simulink model "HVDCThyristorBased"  (R2024b)
settings: Solver=FixedStepDiscrete  StartTime=0.0  StopTime=2  FixedStep=Ts  RelTol=1e-3  AbsTol=1e-2
InitFcn:
  | Ts=50e-6;
  | 
  | % Rectifier AC side :
  | VLL_nom_R = 500e3; % V
  | Fnom_R = 60;           % Hz
  | 
  | % Inverter AC side :
  | VLL_nom_I = 345e3; % V
  | Fnom_I = 50;           % Hz
  | 
  | % DC :
  | Vdc_nom = 500e3;   % V
  | Idc_nom  = 2000;     % A
undefined symbols (not defined in the file or in its folder): D1, Delta, lagging, pulse, test_alpha
libraries: simulink x24, spsOnDelayLib x12, spsFirstOrderFilterLib x9, spsSampleandHoldLib x8, spsMultimeterLib x7, spsMonostableLib x7, spsThreePhaseHarmonicFilterLib x6, spsEdgeDetectorLib x6, spsGroundLib x4, spsUniversalBridgeLib x4, spsImpedanceMeasurementLib x3, spsBistableLib x3
(part 1 of 5)
Description:
  | The 'Model  initialization function' defined in the
  | 
  | Model Properties automatically sets the sample time
  | 
  | Ts to 50e-6 s
settings Model: Creator=The MathWorks, Inc.  LastModifiedBy=prankfarsons
settings SolverCC: AutoScaleAbsTol=off  AlgebraicLoopSolver=TrustRegion
settings DataIOCC: SaveFormat=StructureWithTime  SaveTime=off  ReturnWorkspaceOutputs=off  SignalLoggingName=sigsOut
settings OptimizationCC: BlockReduction=off  BooleanDataType=off  ExpressionDepthLimit=2147483647  InitFltsAndDblsToZero=on  EfficientMapNaN2IntZero=off  LifeSpan=inf
settings DebuggingCC: SaveWithParameterizedLinksMsg=none  UnderspecifiedInitializationDetection=Classic  MergeDetectMultiDrivingBlocksExec=none  CheckExecutionContextPreStartOutputMsg=on  SignalResolutionControl=TryResolveAllWithWarning  MultiTaskDSMMsg=warning  MultiTaskCondExecSysMsg=none  FcnCallInpInsideContextMsg=warning  UnconnectedLineMsg=warning  StateNameClashWarn=warning  SFUnexpectedBacktrackingDiag=warning  SFNoUnconditionalDefaultTransitionDiag=warning  SFExecutionAtInitializationDiag=none  ArithmeticOperatorsInVariantConditions=warning
settings HardwareCC: ProdBitPerPointer=32  ProdBitPerSizeT=32  ProdBitPerPtrDiffT=32  ProdLargestAtomicFloat=None  ProdIntDivRoundTo=Undefined  ProdEndianess=Unspecified  ProdWordSize=32  ProdHWDeviceType=32-bit Generic  TargetHWDeviceType=32-bit Generic  ProdEqTarget=off
settings ModelReferenceCC: EnableRefExpFcnMdlSchedulingChecks=on  PropagateSignalLabelsOutOfModel=off
settings SFSimCC: SimUseLocalCustomCode=off  CustomCodeUndefinedFunction=UseInterfaceOnly
settings RTWCC: RTWUseLocalCustomCode=off  GPUComputeCapability=3.5  DLArmComputeVersion=19.05
settings CodeAppCC: StateflowObjectComments=on
settings GRTTargetCC: TargetFcnLib=ansi_tfl_tmw.mat  TargetLangStandard=C89/C90 (ANSI)  CombineOutputUpdateFcns=off  GRTInterface=on
settings ConfigComp: CovMetricSettings=dw  CovSaveCumulativeToWorkspaceVar=on  CovSaveSingleToWorkspaceVar=on  CovExternalEMLEnable=off  CovSFcnEnable=off
settings SimscapeCC: SimscapeNormalizeSystem=off

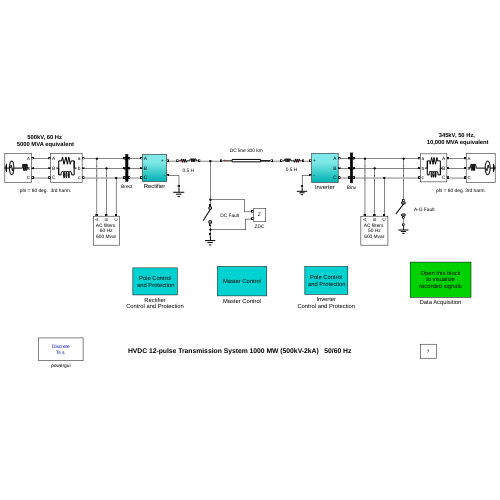
[thumbnail: Simulink's stored preview of the top-level diagram]
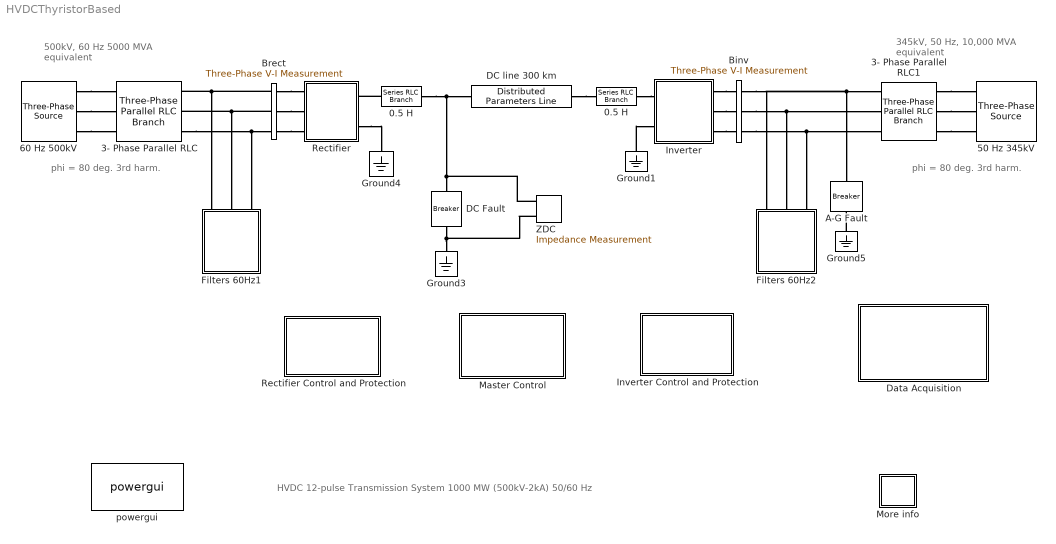
== system HVDCThyristorBased ==
  note: phi = 80 deg. 3rd harm.
  note: HVDC 12-pulse Transmission System 1000 MW (500kV-2kA) 50/60 Hz
  note: 500kV, 60 Hz
      |  5000 MVA equivalent
  note: 345kV, 50 Hz,
      | 10,000 MVA equivalent
  note: phi = 80 deg. 3rd harm.
  " 50 Hz 345kV  " : spsThreePhaseSourceLib/Three-Phase Source  InternalConnection=Yg  VoltagePhases=off  Voltage=VLL_nom_I  PhaseAngle=0  Voltage_phases=[25e3 25e3 25e3]/sqrt(3)  PhaseAngles_phases=[0 -120 +120]  Frequency=Fnom_I  NonIdealSource=on  SpecifyImpedance=off  Resistance=0  Inductance=28.0e-3  ShortCircuitLevel=0  BaseVoltage=0  XRratio=0  BusType=swing  Pref=0  Qref=0  Prefabc=[10e3, 10e3, 10e3]  Qrefabc=[0, 0, 0]  Qmin=-inf  Qmax=inf
  " 60 Hz 500kV" : spsThreePhaseSourceLib/Three-Phase Source  InternalConnection=Yg  VoltagePhases=off  Voltage=VLL_nom_R  PhaseAngle=0  Voltage_phases=[25e3 25e3 25e3]/sqrt(3)  PhaseAngles_phases=[0 -120 +120]  Frequency=Fnom_R  NonIdealSource=on  SpecifyImpedance=off  Resistance=0  Inductance=98.03e-3  ShortCircuitLevel=0  BaseVoltage=0  XRratio=0  BusType=swing  Pref=0  Qref=0  Prefabc=[10e3, 10e3, 10e3]  Qrefabc=[0, 0, 0]  Qmin=-inf  Qmax=inf
  0.5 H : spsSeriesRLCBranchLib/Series RLC Branch  LConnTagsString=__new0  RConnTagsString=__new0  BranchType=RL  Resistance=1  Inductance=0.5  SetiL0=off  InitialCurrent=0  Capacitance=1.0  Setx0=off  InitialVoltage=0  Measurements=None
  "0.5 H " : spsSeriesRLCBranchLib/Series RLC Branch  LConnTagsString=__new0  RConnTagsString=__new0  BranchType=RL  Resistance=1  Inductance=0.5  SetiL0=off  InitialCurrent=0  Capacitance=1.0  Setx0=off  InitialVoltage=0  Measurements=None
  3- Phase Parallel RLC : spsThreePhaseParallelRLCBranchLib/Three-Phase Parallel RLC Branch  LConnTagsString=A|B|C  RConnTagsString=A|B|C  BranchType=RL  Resistance=26.07  Inductance=48.86e-3  Capacitance=1.0  Measurements=None
  3- Phase Parallel RLC1 : spsThreePhaseParallelRLCBranchLib/Three-Phase Parallel RLC Branch  LConnTagsString=A|B|C  RConnTagsString=A|B|C  BranchType=RL  Resistance=6.205  Inductance=13.96e-3  Capacitance=1.0  Measurements=None
  A-G Fault : spsBreakerLib/Breaker  InitialState=0  SwitchingTimes=[ 0.7 0.8]*100  External=off  BreakerResistance=0.01  SnubberResistance=inf  SnubberCapacitance=inf  Measurements=Branch current  MoreParameters=off  NoBreakLoop=off
      settings: AttributesFormatString=\n
  Binv : spsThreePhaseVIMeasurementLib/Three-Phase V-I Measurement  VoltageMeasurement=phase-to-ground  SetLabelV=on  LabelV=Vabc_I  Vpu=on  VpuLL=off  CurrentMeasurement=yes  SetLabelI=on  LabelI=Iabc_I  Ipu=on  Pbase=100e6  Vbase=345e3  OutputType=Magnitude  PhasorSimulation=off  PSBequivalent=0
  Brect : spsThreePhaseVIMeasurementLib/Three-Phase V-I Measurement  VoltageMeasurement=phase-to-ground  SetLabelV=on  LabelV=Vabc_R  Vpu=on  VpuLL=off  CurrentMeasurement=yes  SetLabelI=on  LabelI=Iabc_R  Ipu=on  Pbase=100e6  Vbase=500e3  OutputType=Magnitude  PhasorSimulation=off  PSBequivalent=0
  DC Fault : spsBreakerLib/Breaker  InitialState=0  SwitchingTimes=[0.7 0.75]*100  External=off  BreakerResistance=1  SnubberResistance=inf  SnubberCapacitance=inf  Measurements=Branch current  MoreParameters=off  NoBreakLoop=off
      settings: AttributesFormatString=\n
  DC line 300 km : spsDistributedParametersLineLib/Distributed Parameters Line  Phases=1  Length=300  Frequency=60  Resistance=0.015  Inductance=0.792e-3  Capacitance=14.4e-9  x1=[-0.00105 1.5486758434687e-11;-0.001 1.53358567747392e-11;-0.00095 1.51806860277802e-11;-0.0009 1.50212985315556e-11;-0.00085 1.48577478316252e-11;-0.0008 1.46900886630999e-11;-0.00075 1.45183769320263e-11;-0.0007 1.43426696964279e-11;-0.00065 1.41630251470068e-11;-0.0006 1.39795025875148e-11;-0.00055 1.37921624147985e-11;-0.0005 1.36010660985273e-11;-0.00045 1.34062761606096e-11;-0.0004 1.3207856154305e-11;-0.00035 1.30058706430391e-11;-0.0003 1.28003851789289e-11;-0.00025 1.25914662810252e-11;-0.0002 1.23791814132796e-11;-0.00015 1.21635989622439e-11;-0.0001 1.19447882145089e-11;-5e-05 1.17228193338908e-11]  x2=[-0.00105 1.53172472947485e-11;-0.001 1.51570895334733e-11;-0.00095 1.49926643749384e-11;-0.0009 1.48240275305931e-11;-0.00085 1.46512359331355e-11;-0.0008 1.44743477170203e-11;-0.00075 1.42934221986079e-11;-0.0007 1.4108519855961e-11;-0.00065 1.39197023082953e-11;-0.0006 1.37270322950921e-11;-0.00055 1.353057365488e-11;-0.0005 1.33303913036921e-11;-0.00045 1.3126551213207e-11;-0.0004 1.29191203885806e-11;-0.00035 1.2708166845976e-11;-0.0003 1.24937595898007e-11;-0.00025 1.2275968589656e-11;-0.0002 1.20548647570092e-11;-0.00015 1.18305199215956e-11;-0.0001 1.16030068075569e-11;-5e-05 1.13723990093264e-11]  x3=[-0.00105 7.66936590964101e-14;-0.001 7.62041024371989e-14;-0.00095 7.56924269415155e-14;-0.0009 7.51588022270623e-14;-0.00085 7.46034044901517e-14;-0.0008 7.40264164464096e-14;-0.00075 7.34280272694635e-14;-0.0007 7.28084325276354e-14;-0.00065 7.21678341186606e-14;-0.0006 7.15064402024553e-14;-0.00055 7.0824465131955e-14;-0.0005 7.01221293820484e-14;-0.00045 6.93996594766289e-14;-0.0004 6.86572879137897e-14;-0.00035 6.7895253089188e-14;-0.0003 6.71137992176017e-14;-0.00025 6.63131762527087e-14;-0.0002 6.54936398051114e-14;-0.00015 6.46554510586376e-14;-0.0001 6.37988766849435e-14;-5e-05 6.29241887564479e-14]  x4=[-0.00105 6.60417424443001e-14;-0.001 6.55953117947027e-14;-0.00095 6.51305000859663e-14;-0.0009 6.46474859539062e-14;-0.00085 6.41464532831615e-14;-0.0008 6.3627591138834e-14;-0.00075 6.30910936965875e-14;-0.0007 6.25371601712336e-14;-0.00065 6.19659947438301e-14;-0.0006 6.13778064873171e-14;-0.00055 6.07728092907198e-14;-0.0005 6.01512217819435e-14;-0.00045 5.95132672491894e-14;-0.0004 5.88591735610186e-14;-0.00035 5.81891730850945e-14;-0.0003 5.75035026056304e-14;-0.00025 5.6802403239573e-14;-0.0002 5.60861203515512e-14;-0.00015 5.53549034676203e-14;-0.0001 5.46090061878316e-14;-5e-05 5.3848686097659e-14]  x5=0.00101312980412186  V1=ones(3,3)  V2=ones(3,3)  I1=ones(3,3)  I2=ones(3,3)  nHarmo=1  Measurements=Phase-to-ground voltages  Decoupling=off  VsMag0=0  VrMag0=0  VsAngle0=0  VrAngle0=0  IsMag0=0  IrMag0=0  IsAngle0=0  IrAngle0=0
      settings: AttributesFormatString=\n
  Data Acquisition : Subsystem
      mask Display: disp('Open this block\nto visualize\nrecorded signals')
  Filters 60Hz1 : Subsystem
      mask Display: disp('AC filters \n60 Hz\n600 Mvar')
  Filters 60Hz2 : Subsystem
      mask Display: disp('AC filters \n50 Hz\n600 Mvar')
  Ground{1,3..5} (4 alike) : spsGroundLib/Ground  LConnTagsString=a
  Inverter : Subsystem
  Inverter Control and Protection : Subsystem
      mask Display: disp('Pole Control\n and Protection')
  Master Control : Subsystem
      mask Display: disp('Master Control')
  More info : Subsystem
      settings: OpenFcn="showExample(\"simscapeelectricalsps/HVDCThyristorBasedExample\")"
      mask Display: disp('?')
  Rectifier : Subsystem
  Rectifier Control and Protection : Subsystem
      mask Display: disp('Pole Control\n and Protection')
  ZDC : spsImpedanceMeasurementLib/Impedance Measurement  LConnTagsString=+|-  Factor=1
  powergui : spspowerguiLib/powergui  Priority=2  SimulationMode=Discrete  SampleTime=Ts  frequency=60  Iterations=50  frequencyindice=60  Pbase=100e6  ErrMax=1e-4  UnitsV=kV  UnitsW=MW  buscounter=0  FunctionMessages=off  echomessages=off  EnableUseOfTLC=off  CurrentSourceSwitches=off  DisableSnubberDevices=off  DisableRonSwitches=off  DisableVfSwitches=off  DisplayEquations=off  AutomaticDiscreteSolvers=off  SolverType=Tustin  Interpol=off  ExternalGateDelay=off  methode=off  Ts=0  x0status=blocks  SPID=off  SwTol=0  HookPort=off  NonlinearTolerance=1e-4  nMaxIteration=100  ContinueOnMaxIteration=off  RestoreLinks=warning  ResistiveCurrentMeasurement=off  Frange=[10:2:1500]  Ylog=off  Xlog=off  ShowGrid=off  save=off  variable=ZData  structure=0  ZoomFFT=on  StartTime=0.0  cycles=1  DisplayStyle=off  fundamental=60  FreqAxis=off  MaxFrequency=1000  frequencyindicesteady=1  RmsSteady=1  display=off
  connections:
  DC Fault/RConn1 -- ZDC/LConn2 -- Ground3/LConn1
  " 60 Hz 500kV"/RConn1 -- 3- Phase Parallel RLC/LConn1
  " 60 Hz 500kV"/RConn2 -- 3- Phase Parallel RLC/LConn2
  " 60 Hz 500kV"/RConn3 -- 3- Phase Parallel RLC/LConn3
  Brect/LConn2 -- 3- Phase Parallel RLC/RConn2 -- Filters 60Hz1/LConn2
  3- Phase Parallel RLC/RConn3 -- Brect/LConn3 -- Filters 60Hz1/LConn3
  Brect/LConn1 -- 3- Phase Parallel RLC/RConn1 -- Filters 60Hz1/LConn1
  Inverter/LConn1 -- Binv/RConn1
  Inverter/LConn2 -- Binv/RConn2
  Inverter/LConn3 -- Binv/RConn3
  Brect/RConn1 -- Rectifier/LConn1
  Brect/RConn2 -- Rectifier/LConn2
  Brect/RConn3 -- Rectifier/LConn3
  0.5 H/LConn1 -- Rectifier/RConn1
  DC line 300 km/RConn1 -- "0.5 H "/RConn1
  "0.5 H "/LConn1 -- Inverter/RConn1
  0.5 H/RConn1 -- DC line 300 km/LConn1 -- ZDC/LConn1 -- DC Fault/LConn1
  Ground5/LConn1 -- A-G Fault/RConn1
  Ground1/LConn1 -- Inverter/RConn2
  Rectifier/RConn2 -- Ground4/LConn1
  3- Phase Parallel RLC1/LConn1 -- " 50 Hz 345kV  "/RConn1
  3- Phase Parallel RLC1/LConn2 -- " 50 Hz 345kV  "/RConn2
  3- Phase Parallel RLC1/LConn3 -- " 50 Hz 345kV  "/RConn3
  Binv/LConn1 -- Filters 60Hz2/LConn1 -- A-G Fault/LConn1 -- 3- Phase Parallel RLC1/RConn1
  Binv/LConn2 -- Filters 60Hz2/LConn2 -- 3- Phase Parallel RLC1/RConn2
  Binv/LConn3 -- Filters 60Hz2/LConn3 -- 3- Phase Parallel RLC1/RConn3

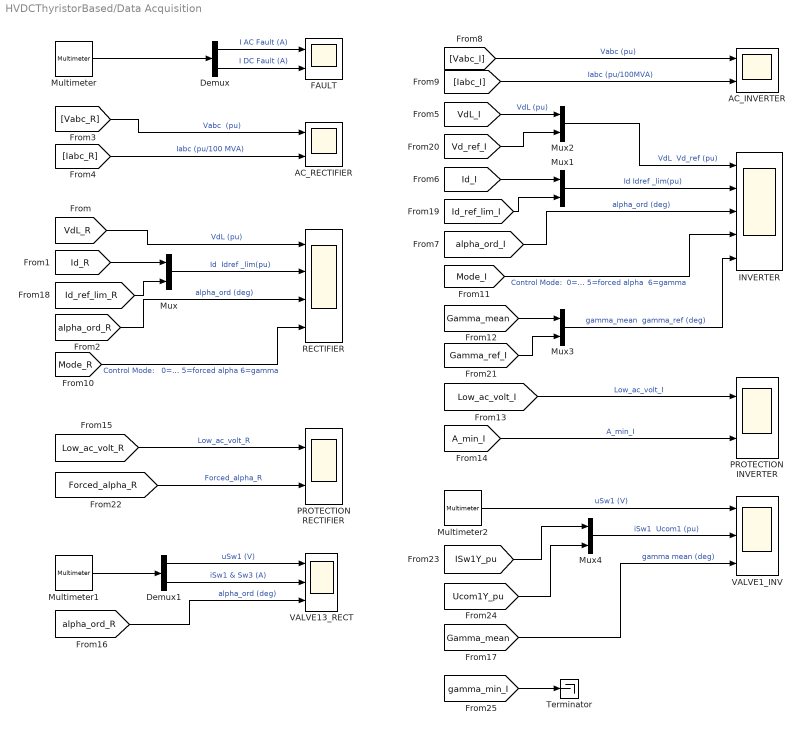
== system HVDCThyristorBased/Data Acquisition ==
  AC_INVERTER : Scope  NumInputPorts=2
  AC_RECTIFIER : Scope  NumInputPorts=2
  Demux : Demux  Outputs=2
      settings: DisplayOption=none
  Demux1 : Demux  Outputs=[1 2]
      settings: DisplayOption=none
  FAULT : Scope  NumInputPorts=2
  INVERTER : Scope  NumInputPorts=5
  Multimeter : spsMultimeterLib/Multimeter  Tag=PoWeRsYsTeMmEaSuReMeNt  L=42  sel=[24 23]  yselected={'Ib: A-G Fault','Ib: DC Fault'};  Gain=[1 1]  OutputType=Magnitude  PlotAtSimulationStop=off  PhasorSimulation=off
      settings: AttributesFormatString=\n
  Multimeter1 : spsMultimeterLib/Multimeter  Tag=PoWeRsYsTeMmEaSuReMeNt  L=42  sel=[11 37 39]  yselected={'Usw1: Rectifier/Rectifier/Bridge Y','Isw1: Rectifier/Rectifier/Bridge Y','Isw3: Rectifier/Rectifier/Bridge Y'};  Gain=[1 1 1]  OutputType=Magnitude  PlotAtSimulationStop=off  PhasorSimulation=off
      settings: AttributesFormatString=\n
  Multimeter2 : spsMultimeterLib/Multimeter  Tag=PoWeRsYsTeMmEaSuReMeNt  L=42  sel=1  yselected={'Usw1: Inverter/Inverter/Bridge Y'};  Gain=1  OutputType=Magnitude  PlotAtSimulationStop=off  PhasorSimulation=off
      settings: AttributesFormatString=\n
  Mux{,1..4} (5 alike) : Mux  Inputs=2
  PROTECTION INVERTER : Scope  NumInputPorts=2
  PROTECTION RECTIFIER : Scope  NumInputPorts=2
  RECTIFIER : Scope  NumInputPorts=4
  Terminator : Terminator
  VALVE13_RECT : Scope  NumInputPorts=3
  VALVE1_INV : Scope  NumInputPorts=3
  wires:
  [Mode_R] -> RECTIFIER/4  "Control Mode:   0=blocked  1=current 2=voltage 3=alpha min  4=alpha max 5=forced alpha 6=gamma"
  Demux/2 -> FAULT/2  "I DC Fault (A)"
  Demux/1 -> FAULT/1  "I AC Fault (A)"
  [alpha_ord_I] -> INVERTER/3  "alpha_ord (deg)"
  [Iabc_I] -> AC_INVERTER/2  "Iabc (pu/100MVA)"
  [Vabc_I] -> AC_INVERTER/1  "Vabc (pu)"
  [alpha_ord_R] -> RECTIFIER/3  "alpha_ord (deg)"
  [VdL_R] -> RECTIFIER/1  "VdL (pu)"
  [Iabc_R] -> AC_RECTIFIER/2  "Iabc (pu/100 MVA)"
  [Vabc_R] -> AC_RECTIFIER/1  "Vabc  (pu)"
  Multimeter/1 -> Demux/1
  [Low_ac_volt_I] -> PROTECTION INVERTER/1  "Low_ac_volt_I"
  [A_min_I] -> PROTECTION INVERTER/2  "A_min_I"
  [Low_ac_volt_R] -> PROTECTION RECTIFIER/1  "Low_ac_volt_R"
  Mux/1 -> RECTIFIER/2  "Id  Idref _lim(pu)"
  [Id_R] -> Mux/1
  [Id_ref_lim_R] -> Mux/2
  [Id_I] -> Mux1/1
  [Id_ref_lim_I] -> Mux1/2
  Mux1/1 -> INVERTER/2  "Id Idref _lim(pu)"
  [Mode_I] -> INVERTER/4  "Control Mode:  0=blocked  1=current  2=voltage  3=alpha min  4=alpha max  5=forced alpha  6=gamma"
  [VdL_I] -> Mux2/1  "VdL (pu)"
  Mux2/1 -> INVERTER/1  "VdL  Vd_ref (pu)"
  [Vd_ref_I] -> Mux2/2
  [Gamma_mean] -> Mux3/1
  Mux3/1 -> INVERTER/5  "gamma_mean  gamma_ref (deg)"
  [Forced_alpha_R] -> PROTECTION RECTIFIER/2  "Forced_alpha_R"
  Multimeter1/1 -> Demux1/1
  Demux1/1 -> VALVE13_RECT/1  "uSw1 (V)"
  Demux1/2 -> VALVE13_RECT/2  "iSw1 & Sw3 (A)"
  [alpha_ord_R] -> VALVE13_RECT/3  "alpha_ord (deg)"
  Multimeter2/1 -> VALVE1_INV/1  "uSw1 (V)"
  Mux4/1 -> VALVE1_INV/2  "iSw1  Ucom1 (pu)"
  [ISw1Y_pu] -> Mux4/1
  [Ucom1Y_pu] -> Mux4/2
  [Gamma_ref_I] -> Mux3/2
  [Gamma_mean] -> VALVE1_INV/3  "gamma mean (deg)"
  [gamma_min_I] -> Terminator/1

== system HVDCThyristorBased/Filters 60Hz1 ==
  note: Capacitor banks
  note: Tuned filters
  note: High-pass
      | damped filter
  note: 60 Hz filters 4*150 Mvars @ 500 kV
  11th 150 Mvar Q=100 : spsThreePhaseHarmonicFilterLib/Three-Phase Harmonic Filter  LConnTagsString=A|B|C  FilterType=Single-tuned  FilterConnection=Y (grounded)  ParNom=[VLL_nom_R, Fnom_R]  Qc=0.25*(Vdc_nom*Idc_nom*0.6)  Fr=[11*Fnom_R]  Frd=[11*60 13*60]  Q=100  Measurements=None
      settings: AttributesFormatString=\n
  "13th 150 Mvar Q=100 " : spsThreePhaseHarmonicFilterLib/Three-Phase Harmonic Filter  LConnTagsString=A|B|C  FilterType=Single-tuned  FilterConnection=Y (grounded)  ParNom=[VLL_nom_R, Fnom_R]  Qc=0.25*(Vdc_nom*Idc_nom*0.6)  Fr=[13*Fnom_R]  Frd=[11*60 13*60]  Q=100  Measurements=None
      settings: AttributesFormatString=\n
  150 Mvar : spsThreePhaseSeriesRLCLoadLib/Three-Phase Series RLC Load  LConnTagsString=A|B|C  Configuration=Y (grounded)  NominalVoltage=VLL_nom_R  Vabc=[1e3 1e3 1e3]  Vabcp=[1e3 1e3 1e3]  NominalFrequency=Fnom_R  UnbalancedPower=off  ActivePower=0  InductivePower=0  CapacitivePower=0.25*(Vdc_nom*Idc_nom*0.6)  Pabc=[10e3 9e3 11e3]  QLabc=[100 90 110]  QCabc=[100 90 110]  Pabcp=[10e3 9e3 11e3]  QLabcp=[100 90 110]  QCabcp=[100 90 110]  Measurements=None  LoadType=constant Z
  24th 150 Mvar Q=3 : spsThreePhaseHarmonicFilterLib/Three-Phase Harmonic Filter  LConnTagsString=A|B|C  FilterType=High-pass  FilterConnection=Y (grounded)  ParNom=[VLL_nom_R, Fnom_R]  Qc=0.25*(Vdc_nom*Idc_nom*0.6)  Fr=[24*Fnom_R]  Frd=[11*60 13*60]  Q=3  Measurements=None
      settings: AttributesFormatString=\n
  A : PMIOPort  Side=Left
  B : PMIOPort  Port=2  Side=Left
  C : PMIOPort  Port=3  Side=Left
  connections:
  150 Mvar/LConn3 -- 24th 150 Mvar Q=3/LConn3 -- "13th 150 Mvar Q=100 "/LConn3 -- 11th 150 Mvar Q=100/LConn3 -- C/RConn1
  150 Mvar/LConn2 -- 24th 150 Mvar Q=3/LConn2 -- "13th 150 Mvar Q=100 "/LConn2 -- 11th 150 Mvar Q=100/LConn2 -- B/RConn1
  150 Mvar/LConn1 -- 24th 150 Mvar Q=3/LConn1 -- "13th 150 Mvar Q=100 "/LConn1 -- 11th 150 Mvar Q=100/LConn1 -- A/RConn1

== system HVDCThyristorBased/Filters 60Hz2 ==
  note: 50 Hz filters 4*150 Mvars @ 345 kV
  note: Tuned filters
  note: Capacitor banks
  note: High-pass
      | damped filter
  11th 150 Mvar Q=100 : spsThreePhaseHarmonicFilterLib/Three-Phase Harmonic Filter  LConnTagsString=A|B|C  FilterType=Single-tuned  FilterConnection=Y (grounded)  ParNom=[VLL_nom_I, Fnom_I]  Qc=0.25*(Vdc_nom*Idc_nom*0.6)  Fr=[11*Fnom_I]  Frd=[11*60 13*60]  Q=100  Measurements=None
      settings: AttributesFormatString=\n
  "13th 150 Mvar Q=100 " : spsThreePhaseHarmonicFilterLib/Three-Phase Harmonic Filter  LConnTagsString=A|B|C  FilterType=Single-tuned  FilterConnection=Y (grounded)  ParNom=[VLL_nom_I, Fnom_I]  Qc=0.25*(Vdc_nom*Idc_nom*0.6)  Fr=[13*Fnom_I]  Frd=[11*60 13*60]  Q=100  Measurements=None
      settings: AttributesFormatString=\n
  150 Mvar : spsThreePhaseSeriesRLCLoadLib/Three-Phase Series RLC Load  LConnTagsString=A|B|C  Configuration=Y (grounded)  NominalVoltage=VLL_nom_I  Vabc=[1e3 1e3 1e3]  Vabcp=[1e3 1e3 1e3]  NominalFrequency=Fnom_I  UnbalancedPower=off  ActivePower=0  InductivePower=0  CapacitivePower=0.25*(Vdc_nom*Idc_nom*0.6)  Pabc=[10e3 9e3 11e3]  QLabc=[100 90 110]  QCabc=[100 90 110]  Pabcp=[10e3 9e3 11e3]  QLabcp=[100 90 110]  QCabcp=[100 90 110]  Measurements=None  LoadType=constant Z
  24th 150 Mvar Q=3 : spsThreePhaseHarmonicFilterLib/Three-Phase Harmonic Filter  LConnTagsString=A|B|C  FilterType=High-pass  FilterConnection=Y (grounded)  ParNom=[VLL_nom_I, Fnom_I]  Qc=0.25*(Vdc_nom*Idc_nom*0.6)  Fr=[24*Fnom_I]  Frd=[11*60 13*60]  Q=3  Measurements=None
      settings: AttributesFormatString=\n
  A : PMIOPort  Side=Left
  B : PMIOPort  Port=2  Side=Left
  C : PMIOPort  Port=3  Side=Left
  connections:
  150 Mvar/LConn1 -- 24th 150 Mvar Q=3/LConn1 -- "13th 150 Mvar Q=100 "/LConn1 -- 11th 150 Mvar Q=100/LConn1 -- A/RConn1
  150 Mvar/LConn2 -- 24th 150 Mvar Q=3/LConn2 -- "13th 150 Mvar Q=100 "/LConn2 -- 11th 150 Mvar Q=100/LConn2 -- B/RConn1
  150 Mvar/LConn3 -- 24th 150 Mvar Q=3/LConn3 -- "13th 150 Mvar Q=100 "/LConn3 -- 11th 150 Mvar Q=100/LConn3 -- C/RConn1

== system HVDCThyristorBased/Inverter ==
  1200 MVA : spsThreePhaseTransformerThreeWindingsLib/Three-Phase Transformer (Three Windings)  Winding1Connection=Yg  Winding2Connection=Y  Winding3Connection=Delta (D1)  CoreType=Three single-phase transformers  SetSaturation=off  Hysteresis=off  DataFile='hysteresis'  SetInitialFlux=off  Measurements=None  UNITS=pu  NominalPower=[ 1200e6 , 50 ]  Winding1="[VLL_nom_I*0.96 0.0025  0 ]"  Winding2="[ 200e3  0.0025 0.24]"  Winding3=[ 200e3 0.0025 0.24 ]  Rm=500  Lm=500  L0=0.5  Saturation="[0 0; 0.0024 1.2; 1.0  1.45]"  InitialFluxes=[-1.10749033878531 0.564800371868647 0.542689966916658]  BreakLoop=off  DiscreteSolver=Trapezoidal iterative  DataType=off  TransfoNumber=0
      settings: AttributesFormatString=\n
  A->pu : Gain  Gain=1/Idc_nom  SaturateOnIntegerOverflow=on  OutDataTypeStr=Inherit: Same as input  ParamDataTypeStr=Inherit: Same as input
  Id : spsCurrentMeasurementLib/Current Measurement  Tag=PoWeRsYsTeMmEaSuReMeNt  PhasorSimulation=off  OutputType=Magnitude  PSBequivalent=0
      settings: AttributesFormatString=\n
  Inverter : Subsystem
      mask Display: plot(0,0,100,100,[30 70 50 30 ], [60 60 40 60], [50 50], [25 40], [50 50], [ 60 75], [30 70], [40 40], [50 60 70], [40 30 30]);
  Zinv : spsImpedanceMeasurementLib/Impedance Measurement  LConnTagsString=+|-  Factor=1/2
  A : PMIOPort  Side=Left
  B : PMIOPort  Port=2  Side=Left
  C : PMIOPort  Port=3  Side=Left
  + : PMIOPort  Port=4  Side=Right
  - : PMIOPort  Port=5  Side=Right
  tag scope: Id_I=global
  wires:
  [PulsesY_I] -> Inverter/1(Py)
  [PulsesD_I] -> Inverter/2(Pd)
  Id/1 -> A->pu/1
  A->pu/1 -> [Id_I]
  connections:
  C/RConn1 -- 1200 MVA/LConn3
  A/RConn1 -- Zinv/LConn1 -- 1200 MVA/LConn1
  -/RConn1 -- Inverter/RConn2
  Inverter/LConn6 -- 1200 MVA/RConn6
  1200 MVA/RConn5 -- Inverter/LConn5
  Inverter/LConn4 -- 1200 MVA/RConn4
  1200 MVA/RConn3 -- Inverter/LConn3
  Inverter/LConn2 -- 1200 MVA/RConn2
  1200 MVA/RConn1 -- Inverter/LConn1
  1200 MVA/LConn2 -- Zinv/LConn2 -- B/RConn1
  +/RConn1 -- Id/LConn1
  Id/RConn1 -- Inverter/RConn1

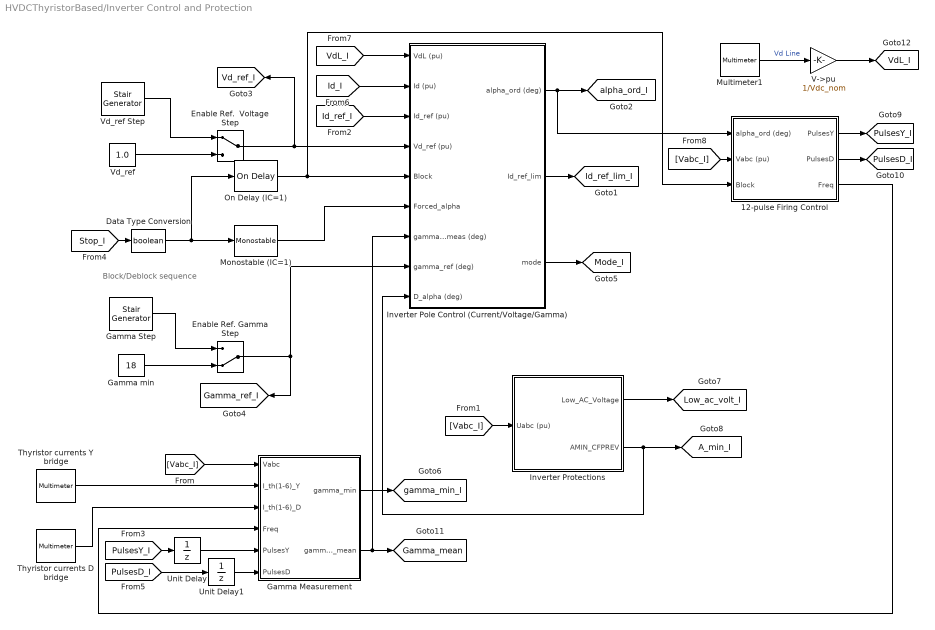
== system HVDCThyristorBased/Inverter Control and Protection ==
  note: Block/Deblock sequence
  12-pulse Firing Control : Subsystem  mask(HVDC Discrete 12-pulse Firing Control){Pw=101.5, PLL_PF=[0,  Fnom_I], PLL_G=[60, 1400], dt=Ts}
      mask prompts: Pw "{Pulse Generator}: Pulse Width (deg)"; PLL_PF "{PLL}: Initial [Phase (deg) Frequency (Hz)]"; PLL_G "{PLL}: Regulator gains [Kp (rad)  Ki (rad/s)]"; dt "Sample Time (s):"
      mask help:
      | This block contains a PLL and a 12-pulse generator to provide the firing pulses to the HVDC converter.
      | The firing control is of the equidistant type. It is based on a Phase Locked Loop (PLL) synchronized on positive-sequence of the fundamental voltage.
      mask init:
      | PLL_ph = PLL_PF(1); PLL_f0 = PLL_PF(2);
      | PLL_Kp = PLL_G(1); PLL_Ki = PLL_G(2);
      mask Help:
      | INPUTS:
      | alpha :  Desired firing angle of thyristors (deg).
      | Vabc  : 3 phase-to-ground voltages (pu)  on the primary winding of the YgYD converter transformer
      | Block  : Logical signal  (0-1). The pulses are not generated when the value is 1.
      | 
      | 
      | 
      | OUTPUTS:
      |  PulsesY :  6 pulses to be sent to the half converter connected to the Wye winding.
      |  PulsesD :  6 pulses to be sent to the half converter connected to the Delta winding.
  Data Type Conversion : DataTypeConversion  OutDataTypeStr=boolean
  Enable Ref.  Voltage Step : ManualSwitch
  Enable Ref. Gamma Step : ManualSwitch  CurrentSetting=0
  Gamma Measurement : Subsystem
  Gamma Step : spsStairGeneratorLib/Stair Generator  t="[ 0  0.7  0.9 ]"  e="[ 18   23   18  ]"  Ts=Ts
  Gamma min : Constant  Value=18
  Inverter Pole Control (Current/Voltage/Gamma) : Subsystem  DialogController=POWERSYS.PowerSysDialog  mask(Discrete HVDC Controller){Mode=Inverter (Current + Voltage + Gamma), XPILim=[166, 92], XLin=[160, 120], XKPI_I=[45, 4500, 90], Id_marg=0.1, XKPI_V=[35, 2250,  90], Vd_marg=0.05, XKPI_G=[2, 40,  90 ], G_marg=1, T_I=0.3e-3, XT_V=[15,  0.707], Xvdcol=[0.6, 0.18, 0.30, 0.1, 0.080], alpha_const=off, Xalpha_fix=[92, inf, -1000], Ts=Ts}
      mask prompts: Mode "Control Mode :"; XPILim "{Alpha Limits}  [alpha max (deg), alpha min (deg) ]"; XLin "Kp Lin. Angle Limits (alpha or beta) : [Max  (deg), Min  (deg) ]"; XKPI_I "{Current Regulator}   [Kp (deg/pu) , Ki (deg/pu/s), AlphaInit (deg) ]"; Id_marg "Current Margin (pu) :"; XKPI_V "{Voltage Regulator}   [Kp (deg/pu) , Ki (deg/pu/s),  AlphaInit (deg) ]"; Vd_marg "Voltage Margin (pu):"; XKPI_G "{Gamma Regulator} [Kp, Ki (s), AlphaInit (deg)]"; G_marg "Gamma Margin (deg):"; T_I "{Id Meas. Filter H(s)=1/(1+Ts)} T(s):"; XT_V "{Vd Meas. Low-Pass 2nd Order Filter}  [fo,  Zeta ]"; Xvdcol "{VDCOL}  [ VdThresh.(pu),VdMin(pu),IdMin(pu),IdMinAbs(pu),Tup(s) ]"; alpha_const "Constant alpha mode"; Xalpha_fix "{Ct.  or Forced alpha)}  [Alpha (deg), + Rate limit, - Rate limit (deg/s)]"; Ts "Sample Time (s):"
      mask help:
      | This block contains the regulators and functions to control the firing angle alpha of a HVDC rectifier or inverter.
      |  See the 'HVDC Transmission System' case study of the User's Manual for description of the block functionality.
      mask init:
      | % Max_lin = max(180-Xlin)  Min_lin = min(180-Xlin)
      | 
      | alpha_max = XPILim(1); alpha_min = XPILim(2);
      | alpha_fix = Xalpha_fix(1); PRate_fix = Xalpha_fix(2);NRate_fix = Xalpha_fix(3);
      | Kp_I = XKPI_I(1); Ki_I = XKPI_I(2); ICi_I = XKPI_I(3);
      | Kp_V = XKPI_V(1); Ki_V = XKPI_V(2); ICi_V = XKPI_V(3);
      | Kp_G = XKPI_G(1); Ki_G = XKPI_G(2); ICi_G = XKPI_G(3);
      | f0_V = XT_V(1); Z_V = XT_V(2);
      | 
      | Inverter = Mode > 1;
      | 
      | if (Mode == 1) 
      | 	Id_marg = 0.0;
      | 	Max_lin = 60; Min_lin = 20;
      | else
      | 	Max_lin = 160; Min_lin = 120;
      | end;
      | 
      | 
      | Vd_seuil = Xvdcol(1); Vd_min=Xvdcol(2);Id_min=Xvdcol(3);Id_min_abs=Xvdcol(4);Tup=Xvdcol(5);
      | if strcmp(alpha_const,'on'), test_alpha = true; else, test_alpha = false; end
      | power_initmask();
      mask Help: This block is part of a subset of blocks in the Extras library that does not have documentation associated with it, other than the block mask description.
      mask TypeOptions Mode: Rectifier (Current) | Inverter (Current + Voltage + Gamma) | Inverter (Current + Voltage) | Inverter (Current + Gamma)
      mask Callback Mode:
      | mode=get_param(gcb,'Mode');
      | 
      | cb=get_param(gcb,'MaskVisibilities');
      | 
      | if strcmp(mode,'Rectifier (Current)')
      | 	cb{10}='on';
      |     cb{11} = 'off';
      | 
      | 	 cb{3}='off';
      | 	 cb{5}='off';cb{6}='off';cb{7}='off';cb{8}='off';cb{9}='off';
      |     set_param(gcb,'MaskVisibilities',cb);
      | elseif (strcmp(mode,'Inverter (Current + Voltage + Gamma)'))
      | 	 cb{3}='off';
      | 	 cb{5}='on';cb{6}='on';cb{7}='on';cb{8}='on';cb{9}='on';cb{11} = 'on';
      | 	 set_param(gcb,'MaskVisibilities',cb);
      | elseif (strcmp(mode,'Inverter (Current + Voltage)'))
      | 	 cb{3}='off';
      | 	 cb{5}='on';cb{6}='on';cb{7}='on';cb{8}='off';cb{9}='off'; cb{11} = 'on';
      |      set_param(gcb,'MaskVisibilities',cb);
      | else
      | 	 cb{3}='off';
      | 	 cb{5}='on';cb{6}='off';cb{7}='off';cb{8}='on';cb{9}='on'; cb{11} = 'on';
      | 	 set_param(gcb,'MaskVisibilities',cb);
      | end
      mask Display: disp('')
  Inverter Protections : Subsystem  TreatAsAtomicUnit=on  mask(Protection LACVD a Radisson (cyc = 1 ms)){}
  Monostable (IC=1) : spsMonostableLib/Monostable  EdgeDetect=Rising  PulseDuration=0.15  ic=1  Ts=Ts
  Multimeter1 : spsMultimeterLib/Multimeter  Tag=PoWeRsYsTeMmEaSuReMeNt  L=42  sel=22  yselected={'Ur_ph1_gnd: DC line 300 km'};  Gain=1  OutputType=Magnitude  PlotAtSimulationStop=off  PhasorSimulation=off
      settings: AttributesFormatString=\n
  On Delay (IC=1) : spsOnDelayLib/On Delay  DelayType=On delay  delay=0.1  ic=1  Ts=Ts
  "Thyristor currents D bridge " : spsMultimeterLib/Multimeter  Tag=PoWeRsYsTeMmEaSuReMeNt  L=42  sel=[25 26 27 28 29 30]  yselected={'Isw1: Inverter/Inverter/Bridge D','Isw2: Inverter/Inverter/Bridge D','Isw3: Inverter/Inverter/Bridge D','Isw4: Inverter/Inverter/Bridge D','Isw5: Inverter/Inverter/Bridge D','Isw6: Inverter/Inverter/Bridge D'};  Gain=[1 1 1 1 1 1]  OutputType=Magnitude  PlotAtSimulationStop=off  PhasorSimulation=off
      settings: AttributesFormatString=\n
  Thyristor currents Y bridge : spsMultimeterLib/Multimeter  Tag=PoWeRsYsTeMmEaSuReMeNt  L=42  sel=[31 32 33 34 35 36]  Gain=[1 1 1 1 1 1]  OutputType=Magnitude  PlotAtSimulationStop=off  PhasorSimulation=off
      settings: AttributesFormatString=\n
  Unit Delay : UnitDelay  SampleTime=Ts  HasFrameUpgradeWarning=on
  Unit Delay1 : UnitDelay  SampleTime=Ts  HasFrameUpgradeWarning=on
  V->pu : Gain  Gain=1/Vdc_nom  SaturateOnIntegerOverflow=on  OutDataTypeStr=Inherit: Same as input  ParamDataTypeStr=Inherit: Same as input
  Vd_ref : Constant  Value=1.0
  Vd_ref Step : spsStairGeneratorLib/Stair Generator  t="[ 0  1  1.2  ]"  e="[ 1   1.1   1  ]"  Ts=Ts
  tag scope: A_min_I=global, Gamma_mean=global, Gamma_ref_I=global, Id_ref_lim_I=global, Low_ac_volt_I=global, Mode_I=global, PulsesD_I=global, PulsesY_I=global, VdL_I=global, Vd_ref_I=global, alpha_ord_I=global, gamma_min_I=global
  wires:
  Data Type Conversion/1 -> On Delay (IC=1)/1, Monostable (IC=1)/1
  [Stop_I] -> Data Type Conversion/1
  [Vabc_I] -> Inverter Protections/1(Uabc (pu))
  Inverter Protections/2(AMIN_CFPREV) -> Inverter Pole Control (Current/Voltage/Gamma)/9(D_alpha (deg)), [A_min_I]
  Inverter Protections/1(Low_AC_Voltage) -> [Low_ac_volt_I]
  V->pu/1 -> [VdL_I]
  Multimeter1/1 -> V->pu/1  "Vd Line"
  Enable Ref. Gamma Step/1 -> Inverter Pole Control (Current/Voltage/Gamma)/8(gamma_ref (deg)), [Gamma_ref_I]
  Gamma Step/1 -> Enable Ref. Gamma Step/1
  Gamma min/1 -> Enable Ref. Gamma Step/2
  Gamma Measurement/1(gamma_min) -> [gamma_min_I]
  [Vabc_I] -> Gamma Measurement/1(Vabc)
  Gamma Measurement/2(gamma_mean) -> Inverter Pole Control (Current/Voltage/Gamma)/7(gamma_meas (deg)), [Gamma_mean]
  Inverter Pole Control (Current/Voltage/Gamma)/1(alpha_ord (deg)) -> 12-pulse Firing Control/1(alpha_ord (deg)), [alpha_ord_I]
  Inverter Pole Control (Current/Voltage/Gamma)/2(Id_ref_lim) -> [Id_ref_lim_I]
  Inverter Pole Control (Current/Voltage/Gamma)/3(mode) -> [Mode_I]
  [Vabc_I] -> 12-pulse Firing Control/2(Vabc (pu))
  [VdL_I] -> Inverter Pole Control (Current/Voltage/Gamma)/1(VdL (pu))
  [Id_I] -> Inverter Pole Control (Current/Voltage/Gamma)/2(Id (pu))
  [Id_ref_I] -> Inverter Pole Control (Current/Voltage/Gamma)/3(Id_ref (pu))
  On Delay (IC=1)/1 -> Inverter Pole Control (Current/Voltage/Gamma)/5(Block), 12-pulse Firing Control/3(Block)
  Enable Ref.  Voltage Step/1 -> Inverter Pole Control (Current/Voltage/Gamma)/4(Vd_ref (pu)), [Vd_ref_I]
  Vd_ref/1 -> Enable Ref.  Voltage Step/2
  Vd_ref Step/1 -> Enable Ref.  Voltage Step/1
  Monostable (IC=1)/1 -> Inverter Pole Control (Current/Voltage/Gamma)/6(Forced_alpha)
  [PulsesD_I] -> Unit Delay1/1
  Thyristor currents Y bridge/1 -> Gamma Measurement/2(I_th(1-6)_Y)
  "Thyristor currents D bridge "/1 -> Gamma Measurement/3(I_th(1-6)_D)
  Unit Delay/1 -> Gamma Measurement/5(PulsesY)
  Unit Delay1/1 -> Gamma Measurement/6(PulsesD)
  [PulsesY_I] -> Unit Delay/1
  12-pulse Firing Control/3(Freq) -> Gamma Measurement/4(Freq)
  12-pulse Firing Control/1(PulsesY) -> [PulsesY_I]
  12-pulse Firing Control/2(PulsesD) -> [PulsesD_I]

== system HVDCThyristorBased/Master Control ==
  note: Master Control
  note: Balanced reference currents
  Constant : Constant  Value=0
  Enable Ref. Current Step : ManualSwitch
  Id_ref Step : spsStairGeneratorLib/Stair Generator  t="[ 0  0.7  0.8  ]"  e="[ 0   -0.2   0  ]"  Ts=Ts
  Informations : Subsystem
      mask Display: disp('?')
  Start/Stop : Subsystem  mask(Start/Stop  & Ramping){Min_ref=0.1, X_start=[0.3333, 0.02], X_up=[5.0, 0.4, 1.0], X_down=[-5.0,  1.4], T_stop=1.6, Ts=Ts}
      mask prompts: Min_ref "Minimum Steady-State Current Reference (pu):"; X_start "{Start Ramp}: [Rate (pu/s), Time (s)]"; X_up "{Up Ramp}: [Rate (pu/s), Time (s), Final Value (pu)]"; X_down "{Down Ramp}: [Rate (-pu/s), Time (s)]"; T_stop "Stop Time (s):"; Ts "Sample Time (s):"
      mask help:
      | At start-up, both converters are deblocked and ramped up to the minimum current (Minimum Steady-State Current Reference) with an adjustable rate (Start Ramp Rate) and application time (Start Ramp Time).
      |
      | After the system stabilisation the current is ramped up to its final value (Up Ramp Final Value) with an adjustable rate (Up Ramp Rate) and execution time (Up Ramp Time).
      |
      | Before stopping the converters (at Stop Time) the current is ramped down to the minimum current  with an adjustable rate (Down Ramp Rate) and execution time  (Down Ramp Time).
      |
      | At Stop Time the reference is ramped down to zero with the same rate used for the Start Ramp.
      mask init:
      | T_up = X_up(2); F_up = X_up(3); up_slope = X_up(1);
      | T_up_final =  T_up + (F_up - Min_ref)/up_slope;
      | 
      | T_down = X_down(2); F_down = Min_ref; down_slope = X_down(1);
      | T_down_final =   T_down + (F_down-F_up)/down_slope;
      | 
      | SS_ramp = X_start(1); T_start = X_start(2);
      | 
      | T_ramp  = [0, T_up, T_up_final,  T_down,  T_down_final, 9999]';
      | U_ramp = [0, 0, F_up-Min_ref,  F_up-Min_ref,  F_down- Min_ref,  F_down - Min_ref]';
      mask Display: disp('Start/Stop\n & Ramping')
  Sum : Sum  SaturateOnIntegerOverflow=on
  tag scope: Id_ref_I=global, Id_ref_R=global, Stop_I=global, Stop_R=global
  wires:
  Id_ref Step/1 -> Enable Ref. Current Step/1
  Constant/1 -> Enable Ref. Current Step/2
  Enable Ref. Current Step/1 -> Sum/2
  Sum/1 -> [Id_ref_R], [Id_ref_I]
  Start/Stop/2("Stop ") -> [Stop_I], [Stop_R]
  Start/Stop/1(Id_ref_ramp) -> Sum/1

== system HVDCThyristorBased/More info ==

== system HVDCThyristorBased/Rectifier ==
  1200 MVA : spsThreePhaseTransformerThreeWindingsLib/Three-Phase Transformer (Three Windings)  Winding1Connection=Yg  Winding2Connection=Y  Winding3Connection=Delta (D1)  CoreType=Three single-phase transformers  SetSaturation=off  Hysteresis=off  DataFile='hysteresis'  SetInitialFlux=off  Measurements=None  UNITS=pu  NominalPower=[ 1200e6 , 60 ]  Winding1="[VLL_nom_R*0.9 0.0025  0 ]"  Winding2=[ 200e3 0.0025 0.24]  Winding3=[ 200e3 0.0025 0.24 ]  Rm=500  Lm=500  L0=0.5  Saturation="[0 0; 0.0024 1.2; 1.0  1.45]"  InitialFluxes=[-1.26114097729929 0.657669801639854 0.603471175659435]  BreakLoop=off  DiscreteSolver=Trapezoidal iterative  DataType=off  TransfoNumber=0
      settings: AttributesFormatString=\n
  A->pu : Gain  Gain=1/Idc_nom  SaturateOnIntegerOverflow=on  OutDataTypeStr=Inherit: Same as input  ParamDataTypeStr=Inherit: Same as input
  Rectifier : Subsystem
      mask Display: plot(0,0,100,100,[30 70 50 30 ], [40 40 60 40], [50 50], [25 40], [50 50], [ 60 75], [30 70], [60 60], [50 40 30], [60 70 70]);
  Zrec : spsImpedanceMeasurementLib/Impedance Measurement  LConnTagsString=+|-  Factor=1/2
  idR : spsCurrentMeasurementLib/Current Measurement  Tag=PoWeRsYsTeMmEaSuReMeNt  PhasorSimulation=off  OutputType=Magnitude  PSBequivalent=0
      settings: AttributesFormatString=\n
  A : PMIOPort  Side=Left
  B : PMIOPort  Port=2  Side=Left
  C : PMIOPort  Port=3  Side=Left
  "+ " : PMIOPort  Port=4  Side=Right
  - : PMIOPort  Port=5  Side=Right
  tag scope: Id_R=global
  wires:
  idR/1 -> A->pu/1
  A->pu/1 -> [Id_R]
  [PulsesY_R] -> Rectifier/1(Py)
  [PulsesD_R] -> Rectifier/2(Pd)
  connections:
  idR/RConn1 -- "+ "/RConn1
  Rectifier/RConn2 -- -/RConn1
  Rectifier/RConn1 -- idR/LConn1
  Rectifier/LConn6 -- 1200 MVA/RConn6
  1200 MVA/RConn5 -- Rectifier/LConn5
  Rectifier/LConn4 -- 1200 MVA/RConn4
  1200 MVA/RConn3 -- Rectifier/LConn3
  Rectifier/LConn2 -- 1200 MVA/RConn2
  1200 MVA/RConn1 -- Rectifier/LConn1
  A/RConn1 -- Zrec/LConn1 -- 1200 MVA/LConn1
  B/RConn1 -- Zrec/LConn2 -- 1200 MVA/LConn2
  C/RConn1 -- 1200 MVA/LConn3

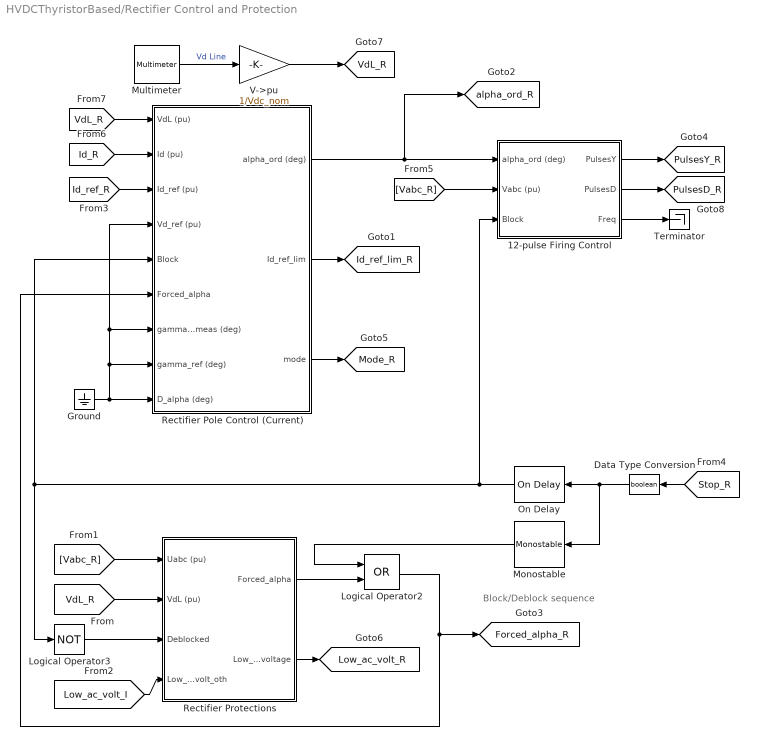
== system HVDCThyristorBased/Rectifier Control and Protection ==
  note: Block/Deblock sequence
  12-pulse Firing Control : Subsystem  mask(HVDC Discrete 12-pulse Firing Control){Pw=101.5, PLL_PF=[0,  Fnom_R], PLL_G=[60, 1400], dt=Ts}
      mask prompts: Pw "{Pulse Generator}: Pulse Width (deg)"; PLL_PF "{PLL}: Initial [Phase (deg) Frequency (Hz)]"; PLL_G "{PLL}: Regulator gains [Kp (rad)  Ki (rad/s)]"; dt "Sample Time (s):"
      mask help:
      | This block contains a PLL and a 12-pulse generator to provide the firing pulses to the HVDC converter.
      | The firing control is of the equidistant type. It is based on a Phase Locked Loop (PLL) synchronized on positive-sequence of the fundamental voltage.
      mask init:
      | PLL_ph = PLL_PF(1); PLL_f0 = PLL_PF(2);
      | PLL_Kp = PLL_G(1); PLL_Ki = PLL_G(2);
      mask Help:
      | INPUTS:
      | alpha :  Desired firing angle of thyristors (deg).
      | Vabc  : 3 phase-to-ground voltages (pu)  on the primary winding of the YgYD converter transformer
      | Block  : Logical signal  (0-1). The pulses are not generated when the value is 1.
      | 
      | 
      | 
      | OUTPUTS:
      |  PulsesY :  6 pulses to be sent to the half converter connected to the Wye winding.
      |  PulsesD :  6 pulses to be sent to the half converter connected to the Delta winding.
  Data Type Conversion : DataTypeConversion  OutDataTypeStr=boolean
  Ground : Ground
  Logical Operator2 : Logic  Operator=OR  AllPortsSameDT=off
  Logical Operator3 : Logic  Operator=NOT
  Monostable : spsMonostableLib/Monostable  EdgeDetect=Rising  PulseDuration=0.15  ic=1  Ts=Ts
  Multimeter : spsMultimeterLib/Multimeter  Tag=PoWeRsYsTeMmEaSuReMeNt  L=42  sel=21  yselected={'Us_ph1_gnd: DC line 300 km'};  Gain=1  OutputType=Magnitude  PlotAtSimulationStop=off  PhasorSimulation=off
      settings: AttributesFormatString=\n
  On Delay : spsOnDelayLib/On Delay  DelayType=On delay  delay=0.1  ic=1  Ts=Ts
  Rectifier Pole Control (Current) : Subsystem  DialogController=POWERSYS.PowerSysDialog  mask(Discrete HVDC Controller){Mode=Rectifier (Current), XPILim=[166, 5], XLin=[160, 120], XKPI_I=[45, 4500, 90], Id_marg=0.1, XKPI_V=[35, 2250,  90], Vd_marg=0.05, XKPI_G=[1, 20,  90 ], G_marg=1, T_I=0.3e-3, XT_V=[15,  0.707], Xvdcol=[0.6, 0.18, 0.30, 0.1, 0.080], alpha_const=off, Xalpha_fix=[166, inf, -inf], Ts=Ts}
      mask prompts: Mode "Control Mode :"; XPILim "{Alpha Limits}  [alpha max (deg), alpha min (deg) ]"; XLin "Kp Lin. Angle Limits (alpha or beta) : [Max  (deg), Min  (deg) ]"; XKPI_I "{Current Regulator}   [Kp (deg/pu) , Ki (deg/pu/s), AlphaInit (deg) ]"; Id_marg "Current Margin (pu) :"; XKPI_V "{Voltage Regulator}   [Kp (deg/pu) , Ki (deg/pu/s),  AlphaInit (deg) ]"; Vd_marg "Voltage Margin (pu):"; XKPI_G "{Gamma Regulator} [Kp, Ki (s), AlphaInit (deg)]"; G_marg "Gamma Margin (deg):"; T_I "{Id Meas. Filter H(s)=1/(1+Ts)} T(s):"; XT_V "{Vd Meas. Low-Pass 2nd Order Filter}  [fo,  Zeta ]"; Xvdcol "{VDCOL}  [ VdThresh.(pu),VdMin(pu),IdMin(pu),IdMinAbs(pu),Tup(s) ]"; alpha_const "Constant alpha mode"; Xalpha_fix "{Ct.  or Forced alpha)}  [Alpha (deg), + Rate limit, - Rate limit (deg/s)]"; Ts "Sample Time (s):"
      mask help:
      | This block contains the regulators and functions to control the firing angle alpha of a HVDC rectifier or inverter.
      |  See the 'HVDC Transmission System' case study of the User's Manual for description of the block functionality.
      mask init: same as HVDCThyristorBased/Inverter Control and Protection/Inverter Pole Control (Current/Voltage/Gamma)
      mask Help: This block is part of a subset of blocks in the Extras library that does not have documentation associated with it, other than the block mask description.
      mask TypeOptions Mode: Rectifier (Current) | Inverter (Current + Voltage + Gamma) | Inverter (Current + Voltage) | Inverter (Current + Gamma)
      mask Callback Mode:
      | mode=get_param(gcb,'Mode');
      | 
      | cb=get_param(gcb,'MaskVisibilities');
      | 
      | if strcmp(mode,'Rectifier (Current)')
      | 	cb{10}='on';
      |     cb{11} = 'off';
      | 
      | 	 cb{3}='off';
      | 	 cb{5}='off';cb{6}='off';cb{7}='off';cb{8}='off';cb{9}='off';
      |     set_param(gcb,'MaskVisibilities',cb);
      | elseif (strcmp(mode,'Inverter (Current + Voltage + Gamma)'))
      | 	 cb{3}='off';
      | 	 cb{5}='on';cb{6}='on';cb{7}='on';cb{8}='on';cb{9}='on';cb{11} = 'on';
      | 	 set_param(gcb,'MaskVisibilities',cb);
      | elseif (strcmp(mode,'Inverter (Current + Voltage)'))
      | 	 cb{3}='off';
      | 	 cb{5}='on';cb{6}='on';cb{7}='on';cb{8}='off';cb{9}='off'; cb{11} = 'on';
      |      set_param(gcb,'MaskVisibilities',cb);
      | else
      | 	 cb{3}='off';
      | 	 cb{5}='on';cb{6}='off';cb{7}='off';cb{8}='on';cb{9}='on'; cb{11} = 'on';
      | 	 set_param(gcb,'MaskVisibilities',cb);
      | end
      mask Display: disp('')
  Rectifier Protections : Subsystem  TreatAsAtomicUnit=on  mask(Protection LACVD a Radisson (cyc = 1 ms)){}
  Terminator : Terminator
  V->pu : Gain  Gain=1/Vdc_nom  SaturateOnIntegerOverflow=on  OutDataTypeStr=Inherit: Same as input  ParamDataTypeStr=Inherit: Same as input
  tag scope: Forced_alpha_R=global, Id_ref_lim_R=global, Low_ac_volt_R=global, Mode_R=global, PulsesD_R=global, PulsesY_R=global, VdL_R=global, alpha_ord_R=global
  wires:
  [Low_ac_volt_I] -> Rectifier Protections/4(Low_ac_volt_oth)
  Rectifier Protections/2(Low_ac_voltage) -> [Low_ac_volt_R]
  Monostable/1 -> Logical Operator2/1
  On Delay/1 -> 12-pulse Firing Control/3(Block), Rectifier Pole Control (Current)/5(Block), Logical Operator3/1
  Rectifier Protections/1(Forced_alpha) -> Logical Operator2/2
  Data Type Conversion/1 -> On Delay/1, Monostable/1
  [Vabc_R] -> Rectifier Protections/1(Uabc (pu))
  [VdL_R] -> Rectifier Protections/2(VdL (pu))
  Logical Operator3/1 -> Rectifier Protections/3(Deblocked)
  [Stop_R] -> Data Type Conversion/1
  Ground/1 -> Rectifier Pole Control (Current)/9(D_alpha (deg)), Rectifier Pole Control (Current)/8(gamma_ref (deg)), Rectifier Pole Control (Current)/7(gamma_meas (deg)), Rectifier Pole Control (Current)/4(Vd_ref (pu))
  [VdL_R] -> Rectifier Pole Control (Current)/1(VdL (pu))
  [Id_R] -> Rectifier Pole Control (Current)/2(Id (pu))
  Rectifier Pole Control (Current)/1(alpha_ord (deg)) -> 12-pulse Firing Control/1(alpha_ord (deg)), [alpha_ord_R]
  Rectifier Pole Control (Current)/2(Id_ref_lim) -> [Id_ref_lim_R]
  Rectifier Pole Control (Current)/3(mode) -> [Mode_R]
  Logical Operator2/1 -> Rectifier Pole Control (Current)/6(Forced_alpha), [Forced_alpha_R]
  Multimeter/1 -> V->pu/1  "Vd Line"
  V->pu/1 -> [VdL_R]
  [Id_ref_R] -> Rectifier Pole Control (Current)/3(Id_ref (pu))
  12-pulse Firing Control/1(PulsesY) -> [PulsesY_R]
  [Vabc_R] -> 12-pulse Firing Control/2(Vabc (pu))
  12-pulse Firing Control/2(PulsesD) -> [PulsesD_R]
  12-pulse Firing Control/3(Freq) -> Terminator/1

== system HVDCThyristorBased/Inverter/Inverter ==
  Py : Inport
  Pd : Inport  Port=2
  Bridge D : spsUniversalBridgeLib/Universal Bridge  Arms=3  SnubberResistance=2000  SnubberCapacitance=0.1e-6  Device=Thyristors  Ron=1e-3  Lon=0  ForwardVoltages="[  0.8  0.8  ]"  ForwardVoltage=0  GTOparameters=[ 10e-6 , 20e-6 ]  IGBTparameters=[ 1e-6 , 2e-6 ]  Measurements=Device currents  Measurements_2=None  converterType=Rectifier
      settings: AttributesFormatString=\n
  Bridge Y : spsUniversalBridgeLib/Universal Bridge  Arms=3  SnubberResistance=2000  SnubberCapacitance=0.1e-6  Device=Thyristors  Ron=1e-3  Lon=0  ForwardVoltages="[  0.8  0.8  ]"  ForwardVoltage=0  GTOparameters=[ 10e-6 , 20e-6 ]  IGBTparameters=[ 1e-6 , 2e-6 ]  Measurements=All voltages and currents  Measurements_2=None  converterType=Rectifier
      settings: AttributesFormatString=\n
  Ay : PMIOPort  Side=Left
  By : PMIOPort  Port=2  Side=Left
  Cy : PMIOPort  Port=3  Side=Left
  Ad : PMIOPort  Port=4  Side=Left
  Bd : PMIOPort  Port=5  Side=Left
  Cd : PMIOPort  Port=6  Side=Left
  pos : PMIOPort  Port=7  Side=Right
  neg : PMIOPort  Port=8  Side=Right
  wires:
  Py/1 -> Bridge Y/1
  Pd/1 -> Bridge D/1
  connections:
  Bridge D/RConn1 -- neg/RConn1
  Bridge Y/RConn2 -- pos/RConn1
  Bridge D/RConn2 -- Bridge Y/RConn1
  Ay/RConn1 -- Bridge Y/LConn1
  By/RConn1 -- Bridge Y/LConn2
  Cy/RConn1 -- Bridge Y/LConn3
  Ad/RConn1 -- Bridge D/LConn1
  Bd/RConn1 -- Bridge D/LConn2
  Cd/RConn1 -- Bridge D/LConn3

== system HVDCThyristorBased/Inverter Control and Protection/12-pulse Firing Control ==
  alpha_ord (deg) : Inport
  Vabc (pu) : Inport  Port=2
  Block : Inport  Port=3
  PLL (3ph) : spsPLL3phLib/PLL (3ph)  Fmin=0.75 * PLL_f0  Par_Init="[PLL_ph  PLL_f0]"  ParK="[PLL_Kp  PLL_Ki  0]"  TcD=1e-4  MaxRateChangeFreq=12  FilterCutOffFreq=25  Ts=Ts  AGC=off
  "Pulse Generator (Thyristor, 12-Pulse)" : spsPulseGeneratorThyristor12PulseLib/Pulse Generator (Thyristor, 12-Pulse)  GenType=12-pulse  Delta=D1 (lagging)  pwidth=Pw  Double_Pulse=off  Ts=Ts
  PulsesY : Outport  VectorParamsAs1DForOutWhenUnconnected=off
  PulsesD : Outport  Port=2  VectorParamsAs1DForOutWhenUnconnected=off
  Freq : Outport  Port=3  VectorParamsAs1DForOutWhenUnconnected=off
  wires:
  Vabc (pu)/1 -> PLL (3ph)/1
  PLL (3ph)/2 -> "Pulse Generator (Thyristor, 12-Pulse)"/2
  alpha_ord (deg)/1 -> "Pulse Generator (Thyristor, 12-Pulse)"/1
  "Pulse Generator (Thyristor, 12-Pulse)"/1 -> PulsesY/1
  "Pulse Generator (Thyristor, 12-Pulse)"/2 -> PulsesD/1
  PLL (3ph)/1 -> Freq/1
  Block/1 -> "Pulse Generator (Thyristor, 12-Pulse)"/3
